simulink model "sedemo_f14_control_over_network"  (Simulink 7.5)
settings: Solver=ode45  SolverMode=SingleTasking  StartTime=0.0  StopTime=100  RelTol=1e-4  AbsTol=1e-6
PreLoadFcn:
  | f14dat
values from neighbouring files (symbols this model uses):
  g = 32.18    [sedemo_absdata.m]
  Kf = 1    [sedemo_absdata.m]
undefined symbols (not defined in the file or in its folder): a, b, des_attributefunction_support, Ka, Ki, Kq, Md, Mq, Mw, Swg, Ta, Tal, Ts, Uo, Vto, W1, W2, Zd, Zw
libraries: simeventsattributes2 x7, simeventssink1 x5, simeventsgenerators1 x5, simeventsrouting1 x4, simulink x3, simeventsqueue1 x3, simeventsinfo x1, simeventstranslate1 x1, simeventssignalmanage1 x1, simeventsserver1 x1
CloseFcn:
  | clear Beta Gamma Ka Kf Ki Kq Md Mq Mw Sa Swg Ta;
  | clear Tal Ts Uo Vto W1 W2 Wa Zd Zw a b cmdgain g;
settings Model: Creator=The MathWorks Inc.  ExtModeTrigMode=oneshot  ExtModeArmWhenConnect=off  ExtModeAutoUpdateStatusClock=off
settings DataIOCC: ExternalInput=[]  InitialState=[]  LimitDataPoints=off  SaveOutput=off  SaveTime=off
settings OptimizationCC: BlockReduction=off  BooleanDataType=off  InitFltsAndDblsToZero=on
settings DebuggingCC: SaveWithParameterizedLinksMsg=none  SignalResolutionControl=TryResolveAllWithWarning  SolverPrmCheckMsg=none  MultiTaskDSMMsg=warning  MultiTaskCondExecSysMsg=none  IntegerOverflowMsg=none  StrictBusMsg=None
settings HardwareCC: TargetUnknown=on
settings RTWCC: IncludeERTFirstTime=on
settings GRTTargetCC: TargetFcnLib=ansi_tfl_tmw.mat
settings SimEventsCC: propDiagAttribOutput=1  propDiagFcnCallOutput=1  propDiagStatOutput=0

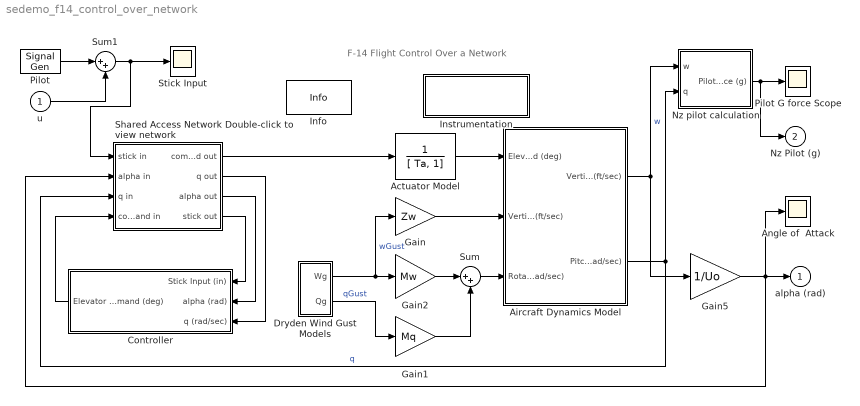
== system sedemo_f14_control_over_network ==
  note: F-14 Flight Control Over a Network
  u : Inport  OutDataType=sfix(16)  OutScaling=2^0
  Actuator Model : TransferFcn  Denominator=[ Ta, 1]
  Aircraft Dynamics Model : Subsystem
  Angle of  Attack : Scope
      settings: TickLabels=on  TimeRange=60  YMin=-1.25  YMax=1.25  DataFormat=Array
  Controller : Subsystem
  Dryden Wind Gust Models : Subsystem
  Gain : Gain  Gain=Zw  ParameterDataType=sfix(16)  ParameterScaling=2^0  OutDataType=sfix(16)  OutScaling=2^0  SaturateOnIntegerOverflow=on  OutDataTypeStr=Inherit: Same as input  ParamDataTypeStr=Inherit: Same as input
  Gain1 : Gain  Gain=Mq  ParameterDataType=sfix(16)  ParameterScaling=2^0  OutDataType=sfix(16)  OutScaling=2^0  SaturateOnIntegerOverflow=on  OutDataTypeStr=Inherit: Same as input  ParamDataTypeStr=Inherit: Same as input
  Gain2 : Gain  Gain=Mw  ParameterDataType=sfix(16)  ParameterScaling=2^0  OutDataType=sfix(16)  OutScaling=2^0  SaturateOnIntegerOverflow=on  OutDataTypeStr=Inherit: Same as input  ParamDataTypeStr=Inherit: Same as input
  Gain5 : Gain  Gain=1/Uo  ParameterDataType=sfix(16)  ParameterScaling=2^0  OutDataType=sfix(16)  OutScaling=2^0  SaturateOnIntegerOverflow=on  OutDataTypeStr=Inherit: Same as input  ParamDataTypeStr=Inherit: Same as input
  Info : simeventsinfo/Info  SystemSampleTime=-1
  Instrumentation : Subsystem
      settings: RequestExecContextInheritance=on
      mask Display: disp('Scopes');
  Nz pilot calculation : Subsystem
  Pilot : SignalGenerator  WaveForm=square  Frequency=0.500000  Units=rad/sec
  Pilot G force Scope : Scope
      settings: TickLabels=on  TimeRange=60  YMin=-15  YMax=15  DataFormat=Array
  Shared Access Network Double-click to view network : Subsystem
  Stick Input : Scope
      settings: TickLabels=on  TimeRange=60  YMin=-1.5  YMax=1.5  DataFormat=Array
  Sum : Sum  Inputs=|++  OutDataType=sfix(16)  OutScaling=2^0  SaturateOnIntegerOverflow=on  InputSameDT=on  OutDataTypeStr=Inherit: Same as first input
  Sum1 : Sum  Inputs=|++  OutDataType=sfix(16)  OutScaling=2^0  SaturateOnIntegerOverflow=on  InputSameDT=on  OutDataTypeStr=Inherit: Same as first input
  alpha (rad) : Outport  OutDataType=sfix(16)  OutScaling=2^0  InitialOutput=0
  Nz Pilot (g) : Outport  Port=2  OutDataType=sfix(16)  OutScaling=2^0  InitialOutput=0
  wires:
  Gain5/1 -> alpha (rad)/1, Angle of  Attack/1, Shared Access Network Double-click to view network/2(alpha in)
  Aircraft Dynamics Model/1(Vertical Velocity w (ft/sec)) -> Gain5/1, Nz pilot calculation/1(w)  "w"
  Nz pilot calculation/1(Pilot g force (g)) -> Pilot G force Scope/1, Nz Pilot (g)/1
  Gain2/1 -> Sum/1
  Gain/1 -> Aircraft Dynamics Model/2(Vertical Gust wGust (ft/sec))
  Pilot/1 -> Sum1/1
  u/1 -> Sum1/2
  Dryden Wind Gust Models/2(Qg) -> Gain1/1  "qGust"
  Dryden Wind Gust Models/1(Wg) -> Gain2/1, Gain/1  "wGust"
  Sum/1 -> Aircraft Dynamics Model/3(Rotary Gust qGust (rad/sec))
  Gain1/1 -> Sum/2
  Aircraft Dynamics Model/2(Pitch Rate q (rad/sec)) -> Nz pilot calculation/2(q), Shared Access Network Double-click to view network/3(q in)  "q"
  Actuator Model/1 -> Aircraft Dynamics Model/1(Elevator Deflection d (deg))
  Sum1/1 -> Stick Input/1, Shared Access Network Double-click to view network/1(stick in)
  Controller/1(Elevator Command (deg)) -> Shared Access Network Double-click to view network/4(command in)
  Shared Access Network Double-click to view network/4(stick out) -> Controller/1(Stick Input (in))
  Shared Access Network Double-click to view network/3(alpha out) -> Controller/2(alpha (rad))
  Shared Access Network Double-click to view network/2(q out) -> Controller/3(q (rad/sec))
  Shared Access Network Double-click to view network/1(command out) -> Actuator Model/1

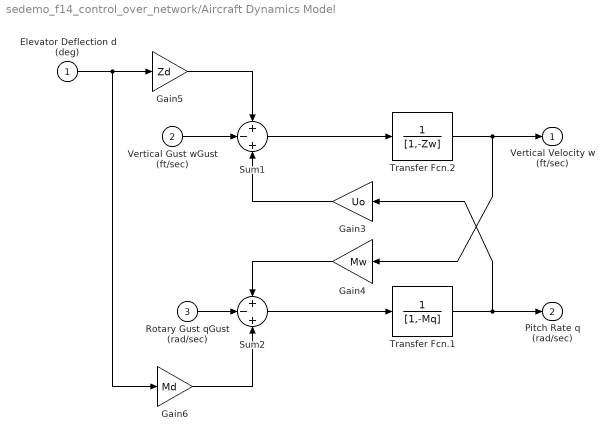
== system sedemo_f14_control_over_network/Aircraft Dynamics Model ==
  Elevator Deflection d (deg) : Inport  OutDataType=sfix(16)  OutScaling=2^0
  Vertical Gust wGust (ft/sec) : Inport  Port=2  OutDataType=sfix(16)  OutScaling=2^0
  Rotary Gust qGust (rad/sec) : Inport  Port=3  OutDataType=sfix(16)  OutScaling=2^0
  Gain3 : Gain  Gain=Uo  ParameterDataType=sfix(16)  ParameterScaling=2^0  OutDataType=sfix(16)  OutScaling=2^0  SaturateOnIntegerOverflow=on  OutDataTypeStr=Inherit: Same as input  ParamDataTypeStr=Inherit: Same as input
  Gain4 : Gain  Gain=Mw  ParameterDataType=sfix(16)  ParameterScaling=2^0  OutDataType=sfix(16)  OutScaling=2^0  SaturateOnIntegerOverflow=on  OutDataTypeStr=Inherit: Same as input  ParamDataTypeStr=Inherit: Same as input
  Gain5 : Gain  Gain=Zd  ParameterDataType=sfix(16)  ParameterScaling=2^0  OutDataType=sfix(16)  OutScaling=2^0  SaturateOnIntegerOverflow=on  OutDataTypeStr=Inherit: Same as input  ParamDataTypeStr=Inherit: Same as input
  Gain6 : Gain  Gain=Md  ParameterDataType=sfix(16)  ParameterScaling=2^0  OutDataType=sfix(16)  OutScaling=2^0  SaturateOnIntegerOverflow=on  OutDataTypeStr=Inherit: Same as input  ParamDataTypeStr=Inherit: Same as input
  Sum1 : Sum  Inputs=+-+  OutDataType=sfix(16)  OutScaling=2^0  SaturateOnIntegerOverflow=on  InputSameDT=on  OutDataTypeStr=Inherit: Same as first input
  Sum2 : Sum  Inputs=+-+  OutDataType=sfix(16)  OutScaling=2^0  SaturateOnIntegerOverflow=on  InputSameDT=on  OutDataTypeStr=Inherit: Same as first input
  Transfer Fcn.1 : TransferFcn  Denominator=[1,-Mq]
  Transfer Fcn.2 : TransferFcn  Denominator=[1,-Zw]
  Vertical Velocity w (ft/sec) : Outport  OutDataType=sfix(16)  OutScaling=2^0  InitialOutput=0
  Pitch Rate q (rad/sec) : Outport  Port=2  OutDataType=sfix(16)  OutScaling=2^0  InitialOutput=0
  wires:
  Transfer Fcn.2/1 -> Vertical Velocity w (ft/sec)/1, Gain4/1
  Transfer Fcn.1/1 -> Pitch Rate q (rad/sec)/1, Gain3/1
  Gain6/1 -> Sum2/3
  Gain5/1 -> Sum1/1
  Gain3/1 -> Sum1/3
  Rotary Gust qGust (rad/sec)/1 -> Sum2/2
  Sum2/1 -> Transfer Fcn.1/1
  Sum1/1 -> Transfer Fcn.2/1
  Gain4/1 -> Sum2/1
  Vertical Gust wGust (ft/sec)/1 -> Sum1/2
  Elevator Deflection d (deg)/1 -> Gain5/1, Gain6/1

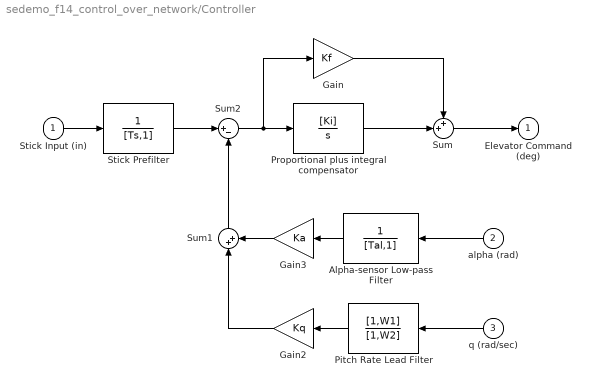
== system sedemo_f14_control_over_network/Controller ==
  Stick Input (in) : Inport  OutDataType=sfix(16)  OutScaling=2^0
  alpha (rad) : Inport  Port=2  OutDataType=sfix(16)  OutScaling=2^0
  q (rad/sec) : Inport  Port=3  OutDataType=sfix(16)  OutScaling=2^0
  Alpha-sensor Low-pass Filter : TransferFcn  Denominator=[Tal,1]
  Gain : Gain  Gain=Kf  ParameterDataType=sfix(16)  ParameterScaling=2^0  OutDataType=sfix(16)  OutScaling=2^0  SaturateOnIntegerOverflow=on  OutDataTypeStr=Inherit: Same as input  ParamDataTypeStr=Inherit: Same as input
  Gain2 : Gain  Gain=Kq  ParameterDataType=sfix(16)  ParameterScaling=2^0  OutDataType=sfix(16)  OutScaling=2^0  SaturateOnIntegerOverflow=on  OutDataTypeStr=Inherit: Same as input  ParamDataTypeStr=Inherit: Same as input
  Gain3 : Gain  Gain=Ka  ParameterDataType=sfix(16)  ParameterScaling=2^0  OutDataType=sfix(16)  OutScaling=2^0  SaturateOnIntegerOverflow=on  OutDataTypeStr=Inherit: Same as input  ParamDataTypeStr=Inherit: Same as input
  Pitch Rate Lead Filter : TransferFcn  Numerator=[1,W1]  Denominator=[1,W2]
  Proportional plus integral compensator : TransferFcn  Numerator=[Ki]  Denominator=[1,0]
  Stick Prefilter : TransferFcn  Denominator=[Ts,1]
  Sum : Sum  Inputs=++|  OutDataType=sfix(16)  OutScaling=2^0  SaturateOnIntegerOverflow=on  InputSameDT=on  OutDataTypeStr=Inherit: Same as first input
  Sum1 : Sum  Inputs=|++  OutDataType=sfix(16)  OutScaling=2^0  SaturateOnIntegerOverflow=on  InputSameDT=on  OutDataTypeStr=Inherit: Same as first input
  Sum2 : Sum  Inputs=|+-  OutDataType=sfix(16)  OutScaling=2^0  SaturateOnIntegerOverflow=on  InputSameDT=on  OutDataTypeStr=Inherit: Same as first input
  Elevator Command (deg) : Outport  OutDataType=sfix(16)  OutScaling=2^0  InitialOutput=0
  wires:
  Sum2/1 -> Proportional plus integral compensator/1, Gain/1
  Gain/1 -> Sum/1
  Proportional plus integral compensator/1 -> Sum/2
  Stick Prefilter/1 -> Sum2/1
  Sum/1 -> Elevator Command (deg)/1
  Gain2/1 -> Sum1/1
  Gain3/1 -> Sum1/2
  Sum1/1 -> Sum2/2
  Pitch Rate Lead Filter/1 -> Gain2/1
  q (rad/sec)/1 -> Pitch Rate Lead Filter/1
  Alpha-sensor Low-pass Filter/1 -> Gain3/1
  alpha (rad)/1 -> Alpha-sensor Low-pass Filter/1
  Stick Input (in)/1 -> Stick Prefilter/1

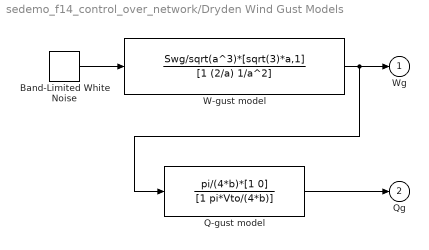
== system sedemo_f14_control_over_network/Dryden Wind Gust Models ==
  Band-Limited White Noise : simulink/Sources/Band-Limited White Noise  SystemSampleTime=-1  Cov=1  Ts=0.1  seed=[23341]
  Q-gust model : TransferFcn  Numerator=pi/(4*b)*[1 0]  Denominator=[1 pi*Vto/(4*b)]
  W-gust model : TransferFcn  Numerator=Swg/sqrt(a^3)*[sqrt(3)*a,1]  Denominator=[1 (2/a) 1/a^2]
  Wg : Outport  OutDataType=sfix(16)  OutScaling=2^0  InitialOutput=0
  Qg : Outport  Port=2  OutDataType=sfix(16)  OutScaling=2^0  InitialOutput=0
  wires:
  Band-Limited White Noise/1 -> W-gust model/1
  Q-gust model/1 -> Qg/1
  W-gust model/1 -> Wg/1, Q-gust model/1

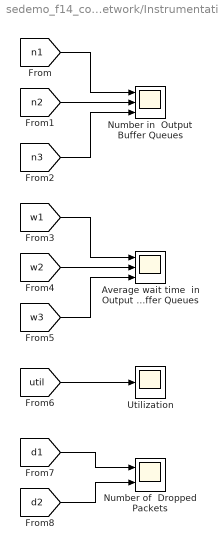
== system sedemo_f14_control_over_network/Instrumentation ==
  Average wait time  in Output Buffer Queues : Scope  NumInputPorts=3
      settings: TimeRange=20  YMin=0~0~0  YMax=0.05~0.05~10  SaveName=ScopeData2  MaxDataPoints=10000  SampleInput=on
  Number in  Output Buffer Queues : Scope  NumInputPorts=3
      settings: TimeRange=10  YMin=0~0~0  YMax=10~10~300  SampleInput=on
  Number of  Dropped Packets : Scope  NumInputPorts=2
      settings: TimeRange=20  YMin=0~0  YMax=200~500  SaveName=ScopeData3  MaxDataPoints=10000  SampleInput=on
  Utilization : Scope
      settings: TimeRange=10  YMin=0  YMax=1.1  SampleInput=on
  wires:
  [n1] -> Number in  Output Buffer Queues/1
  [n2] -> Number in  Output Buffer Queues/2
  [n3] -> Number in  Output Buffer Queues/3
  [w1] -> Average wait time  in Output Buffer Queues/1
  [w2] -> Average wait time  in Output Buffer Queues/2
  [w3] -> Average wait time  in Output Buffer Queues/3
  [util] -> Utilization/1
  [d1] -> Number of  Dropped Packets/1
  [d2] -> Number of  Dropped Packets/2

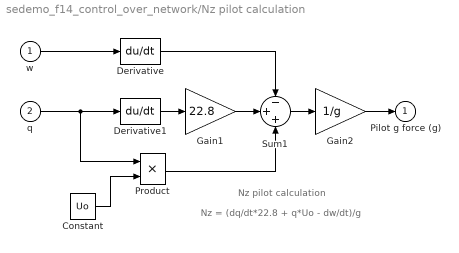
== system sedemo_f14_control_over_network/Nz pilot calculation ==
  note: Nz pilot calculation
  note: Nz = (dq/dt*22.8 + q*Uo - dw/dt)/g
  w : Inport  OutDataType=sfix(16)  OutScaling=2^0
  q : Inport  Port=2  OutDataType=sfix(16)  OutScaling=2^0
  Constant : Constant  Value=Uo  OutDataType=sfix(16)  OutScaling=2^0
  Derivative : Derivative
  Derivative1 : Derivative
  Gain1 : Gain  Gain=22.8  ParameterDataType=sfix(16)  ParameterScaling=2^0  OutDataType=sfix(16)  OutScaling=2^0  SaturateOnIntegerOverflow=on  OutDataTypeStr=Inherit: Same as input  ParamDataTypeStr=Inherit: Same as input
  Gain2 : Gain  Gain=1/g  ParameterDataType=sfix(16)  ParameterScaling=2^0  OutDataType=sfix(16)  OutScaling=2^0  SaturateOnIntegerOverflow=on  OutDataTypeStr=Inherit: Same as input  ParamDataTypeStr=Inherit: Same as input
  Product : Product  OutDataType=sfix(16)  OutScaling=2^0  SaturateOnIntegerOverflow=on  RndMeth=Zero  InputSameDT=on  OutDataTypeStr=Inherit: Same as first input
  Sum1 : Sum  Inputs=-++  OutDataType=sfix(16)  OutScaling=2^0  SaturateOnIntegerOverflow=on  InputSameDT=on  OutDataTypeStr=Inherit: Same as first input
  Pilot g force (g) : Outport  OutDataType=sfix(16)  OutScaling=2^0  InitialOutput=0
  wires:
  q/1 -> Product/1, Derivative1/1
  Constant/1 -> Product/2
  Gain2/1 -> Pilot g force (g)/1
  Sum1/1 -> Gain2/1
  Derivative1/1 -> Gain1/1
  Gain1/1 -> Sum1/2
  Product/1 -> Sum1/3
  Derivative/1 -> Sum1/1
  w/1 -> Derivative/1

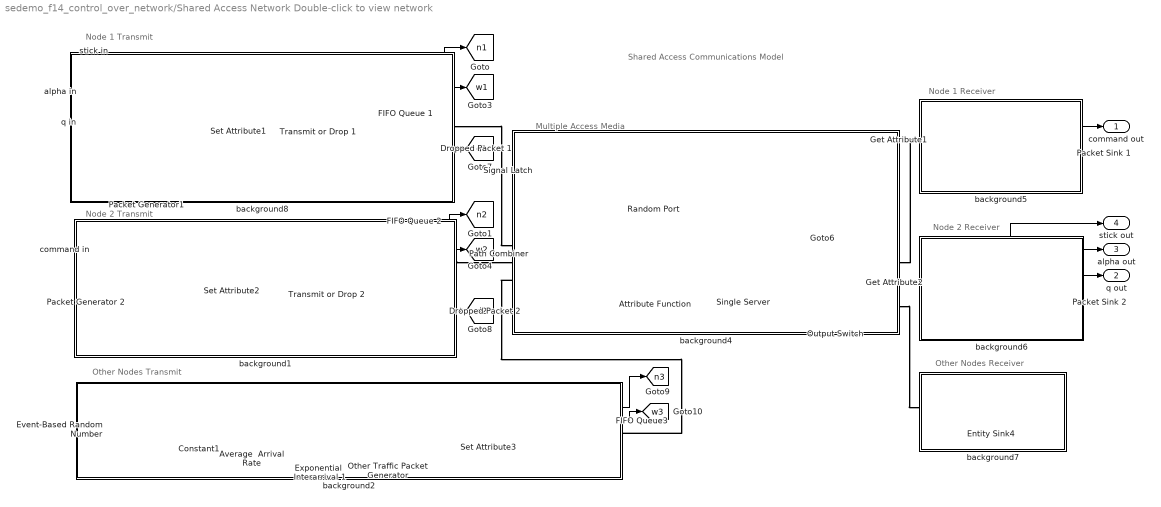
== system sedemo_f14_control_over_network/Shared Access Network Double-click to view network ==
  note: Multiple Access Media
  note: Shared Access Communications Model
  note: Other Nodes Receiver
  note: Node 2 Receiver
  note: Node 1 Receiver
  note: Other Nodes Transmit
  note: Node 2 Transmit
  note: Node 1 Transmit
  stick in : Inport  OutDataType=sfix(16)  OutScaling=2^0
  alpha in : Inport  Port=2  OutDataType=sfix(16)  OutScaling=2^0
  q in : Inport  Port=3  OutDataType=sfix(16)  OutScaling=2^0
  command in : Inport  Port=4  DataType=double  OutDataType=sfix(16)  OutScaling=2^0  OutDataTypeStr=double
  Attribute Function : Subsystem  LoadFcn=des_attributefunction_support(gcb,'LoadFcn');  StartFcn=des_attributefunction_support(gcb,'StartFcn');  mask(Attribute Function){OutputNamePrefix=out_}
      mask prompts: OutputNamePrefix "Prefix name"
      settings: CopyFcn=des_attributefunction_support(gcb,'CopyFcn');  OpenFcn=des_attributefunction_support(gcb,'OpenFcn');  ErrorFcn=des_error_redirect
      mask Display: image(des_iconLoad('attribFunction.jpg'),'center');
  Average  Arrival Rate : simulink/Math Operations/Slider Gain  SystemSampleTime=-1  low=1  gain=124.1935  high=400
  Constant1 : Constant  OutDataType=sfix(16)  OutScaling=2^0
  Dropped Packet 1 : simeventssink1/Entity Sink  Priority=1  SystemSampleTime=-1  AvailableForArrivals=on  StatNumberArrived=On
  Dropped Packet 2 : simeventssink1/Entity Sink  Priority=1  SystemSampleTime=-1  AvailableForArrivals=on  StatNumberArrived=On
  Entity Sink4 : simeventssink1/Entity Sink  Priority=1  SystemSampleTime=-1  AvailableForArrivals=on  StatNumberArrived=Off
  Event-Based Random Number : simeventsgenerators1/Signal Generators/Event-Based Random Number  SystemSampleTime=-1  distribution=Exponential  meanExp=2000  minUnif=0  maxUnif=1  pOneBern=0.25  pSuccessBino=0.5  numTrialBino=1  meanNorm=0  stdNorm=1  minTri=1  maxTri=3  modeTri=2  thresholdLogn=0  scaleLogn=1  shapeLogn=1  pSuccessGeo=0.5  meanPoiss=1  thresholdLogl=0  scaleLogl=1  thresholdGam=0  scaleGam=1  shapeGam=1  minBeta=0  maxBeta=1  shape1Beta=1  shape2Beta=1  minUnid=0  maxUnid=1  numValueUnid=2  thresholdWbl=0  scaleWbl=1  shapeWbl=1  valueVecCont=[0 1]  cdfVecCont=[0 1]  valueVecDisc=[0 1]  probVecDisc=[0.5 0.5]  seed=123457  IsProcessed=on  isConnected=1
  Exponential  Interarrival 1 : Subsystem  mask(Exponential Random Number Generator){rate=0.7, seed=0546269200}
      mask prompts: seed "Initial seed"
      mask help: Generate random numbers with an exponential distribution. User can specify the rate and the initial seed.
      mask Display: plot([0.4 .13 .38 .26 .71 .44 .6 .15 .22 .5 .55 .6 .4]);
  FIFO Queue 1 : simeventsqueue1/FIFO Queue  Priority=1  SystemSampleTime=-1  Capacity=2  EnableTOPort=off  StatNumberDeparted=Off  StatNumberInBlock=On  StatPendingEntity=Off  StatAverageWait=On  StatAverageQueueLength=Off  StatNumberTimedout=Off
  FIFO Queue 2 : simeventsqueue1/FIFO Queue  Priority=1  SystemSampleTime=-1  Capacity=2  EnableTOPort=off  StatNumberDeparted=Off  StatNumberInBlock=On  StatPendingEntity=Off  StatAverageWait=On  StatAverageQueueLength=Off  StatNumberTimedout=Off
  FIFO Queue3 : simeventsqueue1/FIFO Queue  Priority=1  SystemSampleTime=-1  Capacity=200  EnableTOPort=off  StatNumberDeparted=Off  StatNumberInBlock=On  StatPendingEntity=Off  StatAverageWait=On  StatAverageQueueLength=Off  StatNumberTimedout=Off
  Get Attribute1 : simeventsattributes2/Get Attribute  Priority=1  DialogController=des_ddg_create  DialogControllerArgs=DataTag12  SystemSampleTime=-1  AttributeName=Command  AttributeMissing=Error  AttributeDefaultValue=1  AttributeSendTiming=After entity departure  AttributeTreatAsVector=1  StatNumberDeparted=Off  EvaluatedDefaultAttributeValue={[]}
  Get Attribute2 : simeventsattributes2/Get Attribute  Priority=1  DialogController=des_ddg_create  DialogControllerArgs=DataTag14  SystemSampleTime=-1  AttributeName=Stick|Alpha|Q  AttributeMissing=Error|Error|Error  AttributeDefaultValue=1|1|1  AttributeSendTiming=After entity departure|After entity departure|After entity departure  AttributeTreatAsVector=1|1|1  StatNumberDeparted=Off  EvaluatedDefaultAttributeValue={[];[];[]}
  Other Traffic Packet Generator : simeventsgenerators1/Entity Generators/Time-Based Entity Generator  Priority=1  DialogController=des_ddg_create  DialogControllerArgs=DataTag16  SystemSampleTime=-1  GenerateEntitiesUpon=Intergeneration time from port t  Distribution=Uniform  Minimum=0  Maximum=1  Mean=1  InitialSeed=12345  Period=1  PriorityEntityGeneration=1  GenerateEntityAtSimulationStart=on  ResponseWhenBlocked=Pause generation  ResponseWhenUnblocked=Immediate restart  EntityType=Blank  StatNumberDeparted=Off  StatPendingEntity=Off  StatAverageIntergenerationTime=Off
  Output Switch : simeventsrouting1/Output Switch  Priority=1  SystemSampleTime=-1  NumberOutputPorts=3  SwitchingCriterion=From attribute  InitialSeed=34567  AttributeName=DestAddr  InitialConditionsOpt=off  InitialConditions=1  EntityBufferOpt=off  SpecifyEventPriority=off  PriorityOutputSwitchSelectPort=1  TimeoutPortOpt=off  StatNumberDeparted=Off  StatNumberTimedOut=Off  StatPendingEntity=Off  StatLastDeparturePort=Off  EvaluatedNumPorts=3
  Packet Generator 2 : simeventsgenerators1/Entity Generators/Time-Based Entity Generator  Priority=1  DialogController=des_ddg_create  DialogControllerArgs=DataTag19  SystemSampleTime=-1  GenerateEntitiesUpon=Intergeneration time from dialog  Distribution=Constant  Minimum=0  Maximum=1  Mean=1  InitialSeed=123453  Period=0.01  PriorityEntityGeneration=1  GenerateEntityAtSimulationStart=on  ResponseWhenBlocked=Pause generation  ResponseWhenUnblocked=Immediate restart  EntityType=Blank  StatNumberDeparted=Off  StatPendingEntity=Off  StatAverageIntergenerationTime=Off
  Packet Generator1 : simeventsgenerators1/Entity Generators/Time-Based Entity Generator  Priority=1  DialogController=des_ddg_create  DialogControllerArgs=DataTag21  SystemSampleTime=-1  GenerateEntitiesUpon=Intergeneration time from dialog  Distribution=Constant  Minimum=0  Maximum=1  Mean=1  InitialSeed=123457  Period=0.01  PriorityEntityGeneration=1  GenerateEntityAtSimulationStart=on  ResponseWhenBlocked=Pause generation  ResponseWhenUnblocked=Immediate restart  EntityType=Blank  StatNumberDeparted=Off  StatPendingEntity=Off  StatAverageIntergenerationTime=Off
  Packet Sink 1 : simeventssink1/Entity Sink  Priority=1  SystemSampleTime=-1  AvailableForArrivals=on  StatNumberArrived=Off
  Packet Sink 2 : simeventssink1/Entity Sink  Priority=1  SystemSampleTime=-1  AvailableForArrivals=on  StatNumberArrived=Off
  Path Combiner : simeventsrouting1/Path Combiner  Priority=1  SystemSampleTime=-1  NumberInputPorts=3  InputPortPrecedence=From signal port p  InitialSeed=45675  SpecifyEventPriority=off  PriorityPathCombinerPortPrecedenceSelection=4100  StatNumberDeparted=On  StatLastArrivalPort=Off  EvaluatedNumPorts=3
  Random Port : simeventsgenerators1/Signal Generators/Event-Based Random Number  SystemSampleTime=-1  distribution=Arbitrary discrete  meanExp=2000  minUnif=0  maxUnif=1  pOneBern=0.25  pSuccessBino=0.5  numTrialBino=1  meanNorm=0  stdNorm=1  minTri=1  maxTri=3  modeTri=2  thresholdLogn=0  scaleLogn=1  shapeLogn=1  pSuccessGeo=0.5  meanPoiss=1  thresholdLogl=0  scaleLogl=1  thresholdGam=0  scaleGam=1  shapeGam=1  minBeta=0  maxBeta=1  shape1Beta=1  shape2Beta=1  minUnid=0  maxUnid=1  numValueUnid=2  thresholdWbl=0  scaleWbl=1  shapeWbl=1  valueVecCont=[0 1]  cdfVecCont=[0 1]  valueVecDisc=[1 2 3]  probVecDisc=[0.005 0.005 0.990]  seed=123453  IsProcessed=on  isConnected=1
  Set Attribute1 : simeventsattributes2/Set Attribute  Priority=1  DialogController=des_ddg_create  DialogControllerArgs=DataTag26  SystemSampleTime=-1  AttributeFrom=Signal port|Signal port|Signal port|Dialog|Dialog|Dialog  AttributeName=Stick|Alpha|Q|DestAddr|Length|DataRate  AttributeTreatAsVector=1|1|1|1|1|1  AttributeValue=1|1|1|2|2000|1000000  AttributeCreate=on  StatNumberDeparted=Off  EvaluatedAttributeValue={[];[];[];2;2000;1000000}
  Set Attribute2 : simeventsattributes2/Set Attribute  Priority=1  DialogController=des_ddg_create  DialogControllerArgs=DataTag28  SystemSampleTime=-1  AttributeFrom=Dialog|Dialog|Signal port|Dialog  AttributeName=DestAddr|Length|Command|DataRate  AttributeTreatAsVector=1|1|1|1  AttributeValue=1|2000|1|1000000  AttributeCreate=on  StatNumberDeparted=Off  EvaluatedAttributeValue={1;2000;[];1000000}
  Set Attribute3 : simeventsattributes2/Set Attribute  Priority=1  DialogController=des_ddg_create  DialogControllerArgs=DataTag30  SystemSampleTime=-1  AttributeFrom=Dialog|Signal port|Dialog|Dialog  AttributeName=DestAddr|Length|Data|DataRate  AttributeTreatAsVector=1|1|1|1  AttributeValue=3|1|0|1000000  AttributeCreate=on  StatNumberDeparted=Off  EvaluatedAttributeValue={3;[];0;1000000}
  Signal Latch : simeventssignalmanage1/Signal Latch  Priority=1  SystemSampleTime=-1  InitialMemoryValue=1  WriteMemoryUpon=Change in signal from port wvc  MemoryWriteEdgeOption=Rising  SpecifyWriteEventPriority=on  PriorityMemoryWrite=7100  ReadMemoryUpon=Write to memory event  MemoryReadEdgeOption=Falling  SpecifyReadEventPriority=on  PriorityMemoryRead=7000  ReportMemoryState=off  ReportMemoryUponWrite=off  ReportMemoryUponRead=on
  Single Server : simeventsserver1/Single Server  Priority=1  SystemSampleTime=-1  ServiceTimeFrom=Attribute  ServiceTime=0  AttributeName=ServiceTime  PriorityServiceCompletion=500  PermitPreemption=off  SortingAttributeName=PriorityAttributeName  SortingDirection=Ascending  WriteToAttribute=off  ResidualAttributeName=ResidualServiceTime  CreateAttribute=on  EnableTOPort=off  StatNumberDeparted=Off  StatNumberInBlock=Off  StatNumberPreempted=Off  StatPendingEntity=Off  StatAverageWait=Off  StatUtilization=On  StatNumberTimedout=Off
  Transmit or Drop 1 : simeventsrouting1/Output Switch  Priority=1  SystemSampleTime=-1  NumberOutputPorts=2  SwitchingCriterion=First port that is not blocked  InitialSeed=34567  AttributeName=Attribute1  InitialConditionsOpt=off  InitialConditions=1  EntityBufferOpt=off  SpecifyEventPriority=off  PriorityOutputSwitchSelectPort=1  TimeoutPortOpt=off  StatNumberDeparted=Off  StatNumberTimedOut=Off  StatPendingEntity=Off  StatLastDeparturePort=Off  EvaluatedNumPorts=2
  Transmit or Drop 2 : simeventsrouting1/Output Switch  Priority=1  SystemSampleTime=-1  NumberOutputPorts=2  SwitchingCriterion=First port that is not blocked  InitialSeed=34567  AttributeName=Attribute1  InitialConditionsOpt=off  InitialConditions=1  EntityBufferOpt=off  SpecifyEventPriority=off  PriorityOutputSwitchSelectPort=1  TimeoutPortOpt=off  StatNumberDeparted=Off  StatNumberTimedOut=Off  StatPendingEntity=Off  StatLastDeparturePort=Off  EvaluatedNumPorts=2
  background1 : Subsystem
      mask Display: disp('')
  background2 : Subsystem
      mask Display: disp('')
  background4 : Subsystem
      mask Display: disp('')
  background5 : Subsystem
      mask Display: disp('')
  background6 : Subsystem
      mask Display: disp('')
  background7 : Subsystem
      mask Display: disp('')
  background8 : Subsystem
      mask Display: disp('')
  command out : Outport  OutDataType=sfix(16)  OutScaling=2^0
  q out : Outport  Port=2  OutDataType=sfix(16)  OutScaling=2^0
  alpha out : Outport  Port=3  OutDataType=sfix(16)  OutScaling=2^0
  stick out : Outport  Port=4  OutDataType=sfix(16)  OutScaling=2^0
  tag scope: d1=global, d2=global, n1=global, n2=global, n3=global, util=global, w1=global, w2=global, w3=global
  wires:
  Path Combiner/1 -> Signal Latch/1
  Random Port/1 -> Signal Latch/2
  Exponential  Interarrival 1/1(Out1) -> Other Traffic Packet Generator/1
  Average  Arrival Rate/1 -> Exponential  Interarrival 1/1(rate)
  Constant1/1 -> Average  Arrival Rate/1
  Event-Based Random Number/1 -> Set Attribute3/1
  FIFO Queue3/2 -> [w3]
  FIFO Queue3/1 -> [n3]
  Get Attribute2/3 -> q out/1
  Get Attribute2/2 -> alpha out/1
  Get Attribute2/1 -> stick out/1
  q in/1 -> Set Attribute1/3
  alpha in/1 -> Set Attribute1/2
  stick in/1 -> Set Attribute1/1
  Signal Latch/1 -> Path Combiner/1
  FIFO Queue 2/1 -> [n2]
  FIFO Queue 2/2 -> [w2]
  Dropped Packet 2/1 -> [d2]
  Dropped Packet 1/1 -> [d1]
  command in/1 -> Set Attribute2/1
  Single Server/1 -> [util]
  Get Attribute1/1 -> command out/1
  FIFO Queue 1/2 -> [w1]
  FIFO Queue 1/1 -> [n1]
  connections:
  FIFO Queue 1/LConn1 -- Transmit or Drop 1/RConn1
  Transmit or Drop 1/LConn1 -- Set Attribute1/RConn1
  Other Traffic Packet Generator/RConn1 -- Set Attribute3/LConn1
  FIFO Queue 2/RConn1 -- Path Combiner/LConn2
  Output Switch/RConn3 -- Entity Sink4/LConn1
  Get Attribute1/RConn1 -- Packet Sink 1/LConn1
  FIFO Queue 1/RConn1 -- Path Combiner/LConn1
  Set Attribute3/RConn1 -- FIFO Queue3/LConn1
  Path Combiner/LConn3 -- FIFO Queue3/RConn1
  Packet Generator1/RConn1 -- Set Attribute1/LConn1
  Get Attribute2/RConn1 -- Packet Sink 2/LConn1
  Single Server/RConn1 -- Output Switch/LConn1
  Attribute Function/LConn1 -- Path Combiner/RConn1
  Transmit or Drop 1/RConn2 -- Dropped Packet 1/LConn1
  Transmit or Drop 2/RConn2 -- Dropped Packet 2/LConn1
  Transmit or Drop 2/RConn1 -- FIFO Queue 2/LConn1
  Output Switch/RConn1 -- Get Attribute1/LConn1
  Set Attribute2/RConn1 -- Transmit or Drop 2/LConn1
  Packet Generator 2/RConn1 -- Set Attribute2/LConn1
  Get Attribute2/LConn1 -- Output Switch/RConn2
  Attribute Function/RConn1 -- Single Server/LConn1

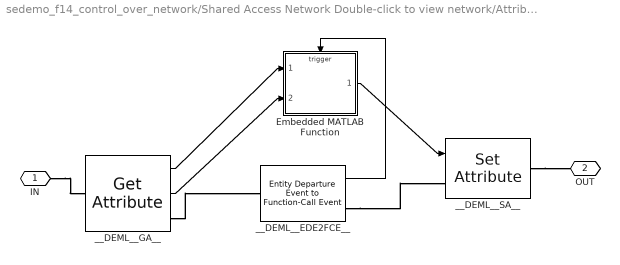
== system sedemo_f14_control_over_network/Shared Access Network Double-click to view network/Attribute Function ==
  Embedded MATLAB Function : Stateflow chart  TreatAsAtomicUnit=on
      settings: PropExecContextOutsideSubsystem=on
  __DEML__EDE2FCE__ : simeventstranslate1/Entity Departure Event to Function-Call Event  Priority=1  SystemSampleTime=-1  TimingFunctionCallF1=Before entity departure  EnableE1Port=off  EnableF2Port=off  TimingFunctionCallF2=Before entity departure  EnableE2Port=off  StatNumberDeparted=Off  StatNumberF1Calls=Off  StatNumberF2Calls=Off  IsInsideAFB=on
  __DEML__GA__ : simeventsattributes2/Get Attribute  Priority=1  DialogController=des_ddg_create  DialogControllerArgs=DataTag2  SystemSampleTime=-1  AttributeName=Length|DataRate  AttributeMissing=Error|Error  AttributeDefaultValue=1|1  AttributeSendTiming=Before entity departure|Before entity departure  AttributeTreatAsVector=1|1  StatNumberDeparted=Off  EvaluatedDefaultAttributeValue={[];[]}
  __DEML__SA__ : simeventsattributes2/Set Attribute  Priority=1  DialogController=des_ddg_create  DialogControllerArgs=DataTag4  SystemSampleTime=-1  AttributeFrom=Signal port  AttributeName=ServiceTime  AttributeTreatAsVector=1  AttributeValue=1  AttributeCreate=on  StatNumberDeparted=Off  EvaluatedAttributeValue={[]}
  IN : PMIOPort  Port=1  Side=Left
  OUT : PMIOPort  Port=2  Side=Right
  wires:
  __DEML__EDE2FCE__/1 -> Embedded MATLAB Function/Trigger
  __DEML__GA__/1 -> Embedded MATLAB Function/1(Length)
  __DEML__GA__/2 -> Embedded MATLAB Function/2(DataRate)
  Embedded MATLAB Function/1(out_ServiceTime) -> __DEML__SA__/1
  connections:
  __DEML__SA__/RConn1 -- OUT/RConn1
  IN/RConn1 -- __DEML__GA__/LConn1
  __DEML__GA__/RConn1 -- __DEML__EDE2FCE__/LConn1
  __DEML__EDE2FCE__/RConn1 -- __DEML__SA__/LConn1

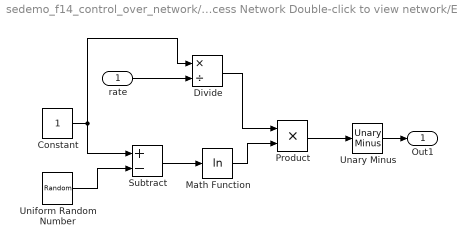
== system sedemo_f14_control_over_network/Shared Access Network Double-click to view network/Exponential  Interarrival 1 ==
  rate : Inport  OutDataType=sfix(16)  OutScaling=2^0
  Constant : Constant  OutDataType=sfix(16)  OutScaling=2^0
  Divide : Product  Inputs=*/  OutDataType=sfix(16)  OutScaling=2^-10
  Math Function : Math  Operator=log  OutDataType=sfix(16)  OutScaling=2^0  SaturateOnIntegerOverflow=on
  Product : Product  OutDataType=sfix(16)  OutScaling=2^0  RndMeth=Zero
  Subtract : Sum  Inputs=+-  OutDataType=sfix(16)  OutScaling=2^-10
  Unary Minus : simulink/Math Operations/Unary Minus  DoSatur=off
  Uniform Random Number : UniformRandomNumber  Minimum=0  Seed=seed  SampleTime=0
  Out1 : Outport  OutDataType=sfix(16)  OutScaling=2^0
  wires:
  Divide/1 -> Product/1
  rate/1 -> Divide/2
  Constant/1 -> Divide/1, Subtract/1
  Uniform Random Number/1 -> Subtract/2
  Subtract/1 -> Math Function/1
  Math Function/1 -> Product/2
  Product/1 -> Unary Minus/1
  Unary Minus/1 -> Out1/1

== system sedemo_f14_control_over_network/Shared Access Network Double-click to view network/background1 ==

== system sedemo_f14_control_over_network/Shared Access Network Double-click to view network/background2 ==

== system sedemo_f14_control_over_network/Shared Access Network Double-click to view network/background4 ==

== system sedemo_f14_control_over_network/Shared Access Network Double-click to view network/background5 ==

== system sedemo_f14_control_over_network/Shared Access Network Double-click to view network/background6 ==

== system sedemo_f14_control_over_network/Shared Access Network Double-click to view network/background7 ==

== system sedemo_f14_control_over_network/Shared Access Network Double-click to view network/background8 ==

== matlab function Shared Access Network Double-click to view network/Attribute Function/Embedded MATLAB Function ==
  data: Length input double; out_ServiceTime output double; DataRate input double
  events: trigger input FUNCTION_CALL_EVENT
function out_ServiceTime  = fcn(Length,DataRate)

out_ServiceTime = Length/DataRate;
